simulink model "ServoControlWSpeed_x10"  (R2014a)
settings: Solver=FixedStepDiscrete  StartTime=0.0  StopTime=400000  FixedStep=1  RelTol=1e-3
libraries: hdlsllib x18, simulink x2
settings Model: Creator=schirner  LastModifiedBy=rouan.c
settings DataIOCC: SaveFormat=StructureWithTime
settings OptimizationCC: BlockReduction=off  ConditionallyExecuteInputs=off  InlineParams=on
settings DebuggingCC: AlgebraicLoopMsg=error  MergeDetectMultiDrivingBlocksExec=error
settings HardwareCC: ProdHWDeviceType=ASIC/FPGA->ASIC/FPGA  ProdEqTarget=off

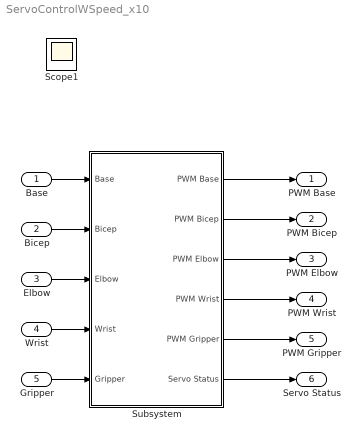
== system ServoControlWSpeed_x10 ==
  Base : Inport  OutDataTypeStr=uint16  SampleTime=1
  Bicep : Inport  Port=2  OutDataTypeStr=uint16  SampleTime=1
  Elbow : Inport  Port=3  OutDataTypeStr=uint16  SampleTime=1
  Wrist : Inport  Port=4  OutDataTypeStr=uint16  SampleTime=1
  Gripper : Inport  Port=5  OutDataTypeStr=uint16  SampleTime=1
  Subsystem : Subsystem  TreatAsAtomicUnit=on  SystemSampleTime=1
  PWM Base : Outport
  PWM Bicep : Outport  Port=2
  PWM Elbow : Outport  Port=3
  PWM Wrist : Outport  Port=4
  PWM Gripper : Outport  Port=5
  Servo Status : Outport  Port=6
  Scope1 : Scope
  wires:
  Subsystem/1(PWM Base) -> PWM Base/1
  Subsystem/2(PWM Bicep) -> PWM Bicep/1
  Subsystem/3(PWM Elbow) -> PWM Elbow/1
  Subsystem/4(PWM Wrist) -> PWM Wrist/1
  Subsystem/5(PWM Gripper) -> PWM Gripper/1
  Subsystem/6("Servo Status ") -> Servo Status/1
  Elbow/1 -> Subsystem/3(Elbow)
  Wrist/1 -> Subsystem/4(Wrist)
  Gripper/1 -> Subsystem/5(Gripper)
  Base/1 -> Subsystem/1(Base)
  Bicep/1 -> Subsystem/2(Bicep)

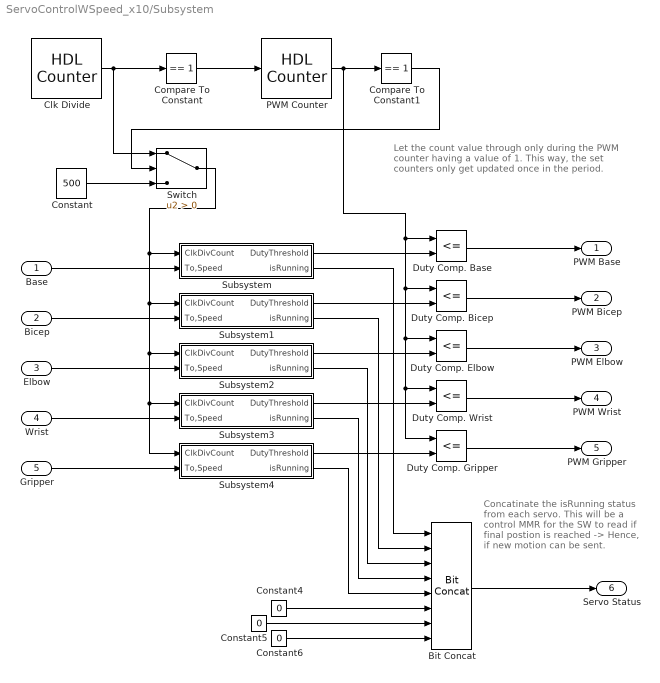
== system ServoControlWSpeed_x10/Subsystem ==
  note: Let the count value through only during
      | the PWM counter having a value of 1.
      | This way, the set counters only get updated
      | once in the period.
  note: Concatinate the isRunning status from each servo. This will be a control MMR for the SW to read if final postion is reached -> Hence, if new motion can be sent.
  Base : Inport  OutDataTypeStr=uint16
  Bicep : Inport  Port=2  OutDataTypeStr=uint16
  Elbow : Inport  Port=3  OutDataTypeStr=uint16
  Wrist : Inport  Port=4  OutDataTypeStr=uint16
  Gripper : Inport  Port=5  OutDataTypeStr=uint16
  Bit Concat : hdlsllib/HDL Operations/Bit Concat  numInputs=8
  Clk Divide : hdlsllib/HDL Operations/HDL Counter  CountType=Count limited  CountInit=1  CountStep=1  CountMax=50  CountFromType=Initial value  CountFrom=1  CountResetPort=off  CountLoadPort=off  CountEnbPort=off  CountDirPort=off  CountDataType=Unsigned  CountWordLen=16  CountFracLen=0  CountSampTime=1
  Compare To Constant : simulink/Logic and Bit Operations/Compare To Constant  relop===  const=1  OutDataTypeStr=boolean
  Compare To Constant1 : simulink/Logic and Bit Operations/Compare To Constant  relop===  const=1  OutDataTypeStr=boolean
  Constant : Constant  Value=500  OutDataTypeStr=int16
  Constant4 : Constant  Value=0  OutDataTypeStr=boolean
  Constant5 : Constant  Value=0  OutDataTypeStr=boolean
  Constant6 : Constant  Value=0  OutDataTypeStr=boolean
  Duty Comp. Base : RelationalOperator  Operator=<=  OutDataTypeStr=boolean
  Duty Comp. Bicep : RelationalOperator  Operator=<=  OutDataTypeStr=boolean
  Duty Comp. Elbow : RelationalOperator  Operator=<=  OutDataTypeStr=boolean
  Duty Comp. Gripper : RelationalOperator  Operator=<=  OutDataTypeStr=boolean
  Duty Comp. Wrist : RelationalOperator  Operator=<=  OutDataTypeStr=boolean
  PWM Counter : hdlsllib/HDL Operations/HDL Counter  CountType=Count limited  CountInit=1  CountStep=1  CountMax=20000  CountFromType=Initial value  CountFrom=1  CountResetPort=off  CountLoadPort=off  CountEnbPort=on  CountDirPort=off  CountDataType=Unsigned  CountWordLen=16  CountFracLen=0  CountSampTime=1
  Subsystem : Subsystem
  Subsystem1 : Subsystem
  Subsystem2 : Subsystem
  Subsystem3 : Subsystem
  Subsystem4 : Subsystem
  Switch : Switch  Criteria=u2 > Threshold
  PWM Base : Outport
  PWM Bicep : Outport  Port=2
  PWM Elbow : Outport  Port=3
  PWM Wrist : Outport  Port=4
  PWM Gripper : Outport  Port=5
  "Servo Status " : Outport  Port=6  OutDataTypeStr=uint8
  wires:
  Duty Comp. Bicep/1 -> PWM Bicep/1
  Compare To Constant/1 -> PWM Counter/1
  Duty Comp. Elbow/1 -> PWM Elbow/1
  Duty Comp. Gripper/1 -> PWM Gripper/1
  Duty Comp. Wrist/1 -> PWM Wrist/1
  PWM Counter/1 -> Duty Comp. Bicep/1, Duty Comp. Gripper/1, Duty Comp. Wrist/1, Duty Comp. Elbow/1, Duty Comp. Base/1, Compare To Constant1/1
  Duty Comp. Base/1 -> PWM Base/1
  Base/1 -> Subsystem/2(To,Speed)
  Subsystem/1(DutyThreshold) -> Duty Comp. Base/2
  Bit Concat/1 -> "Servo Status "/1
  Subsystem/2(isRunning) -> Bit Concat/1
  Constant6/1 -> Bit Concat/8
  Constant5/1 -> Bit Concat/7
  Constant4/1 -> Bit Concat/6
  Bicep/1 -> Subsystem1/2(To,Speed)
  Elbow/1 -> Subsystem2/2(To,Speed)
  Wrist/1 -> Subsystem3/2(To,Speed)
  Gripper/1 -> Subsystem4/2(To,Speed)
  Subsystem1/1(DutyThreshold) -> Duty Comp. Bicep/2
  Subsystem2/1(DutyThreshold) -> Duty Comp. Elbow/2
  Subsystem3/1(DutyThreshold) -> Duty Comp. Wrist/2
  Subsystem4/1(DutyThreshold) -> Duty Comp. Gripper/2
  Subsystem1/2(isRunning) -> Bit Concat/2
  Subsystem2/2(isRunning) -> Bit Concat/3
  Subsystem3/2(isRunning) -> Bit Concat/4
  Subsystem4/2(isRunning) -> Bit Concat/5
  Compare To Constant1/1 -> Switch/2
  Clk Divide/1 -> Switch/1, Compare To Constant/1
  Constant/1 -> Switch/3
  Switch/1 -> Subsystem1/1(ClkDivCount), Subsystem2/1(ClkDivCount), Subsystem4/1(ClkDivCount), Subsystem3/1(ClkDivCount), Subsystem/1(ClkDivCount)

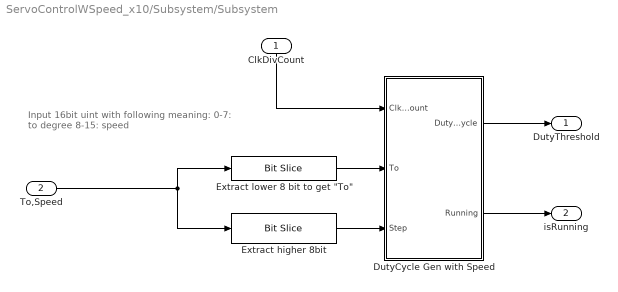
== system ServoControlWSpeed_x10/Subsystem/Subsystem ==
  note: Input 16bit uint with following meaning:
      | 0-7:	to degree
      | 8-15:	speed
  ClkDivCount : Inport
  To,Speed : Inport  Port=2
  DutyCycle Gen with Speed : Subsystem
  Extract higher 8bit : hdlsllib/HDL Operations/Bit Slice  lidx=15  ridx=8
  "Extract lower 8 bit to get \"To\"" : hdlsllib/HDL Operations/Bit Slice  lidx=7  ridx=0
  DutyThreshold : Outport
  isRunning : Outport  Port=2
  wires:
  "Extract lower 8 bit to get \"To\""/1 -> DutyCycle Gen with Speed/2(To)
  ClkDivCount/1 -> DutyCycle Gen with Speed/1(ClkDivCount)
  DutyCycle Gen with Speed/1(Duty Cycle) -> DutyThreshold/1
  To,Speed/1 -> "Extract lower 8 bit to get \"To\""/1, Extract higher 8bit/1
  Extract higher 8bit/1 -> DutyCycle Gen with Speed/3(Step)
  DutyCycle Gen with Speed/2(Running) -> isRunning/1

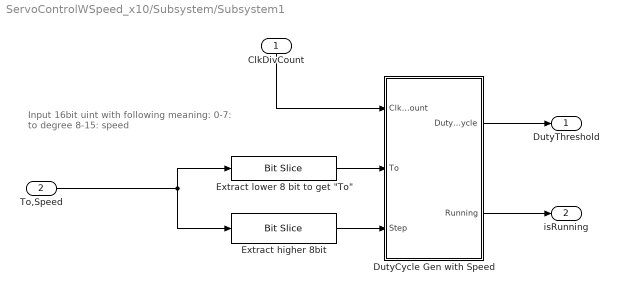
== system ServoControlWSpeed_x10/Subsystem/Subsystem1 ==
  note: Input 16bit uint with following meaning:
      | 0-7:	to degree
      | 8-15:	speed
  ClkDivCount : Inport
  To,Speed : Inport  Port=2
  DutyCycle Gen with Speed : Subsystem
  Extract higher 8bit : hdlsllib/HDL Operations/Bit Slice  lidx=15  ridx=8
  "Extract lower 8 bit to get \"To\"" : hdlsllib/HDL Operations/Bit Slice  lidx=7  ridx=0
  DutyThreshold : Outport
  isRunning : Outport  Port=2
  wires:
  "Extract lower 8 bit to get \"To\""/1 -> DutyCycle Gen with Speed/2(To)
  ClkDivCount/1 -> DutyCycle Gen with Speed/1(ClkDivCount)
  DutyCycle Gen with Speed/1(Duty Cycle) -> DutyThreshold/1
  To,Speed/1 -> "Extract lower 8 bit to get \"To\""/1, Extract higher 8bit/1
  Extract higher 8bit/1 -> DutyCycle Gen with Speed/3(Step)
  DutyCycle Gen with Speed/2(Running) -> isRunning/1

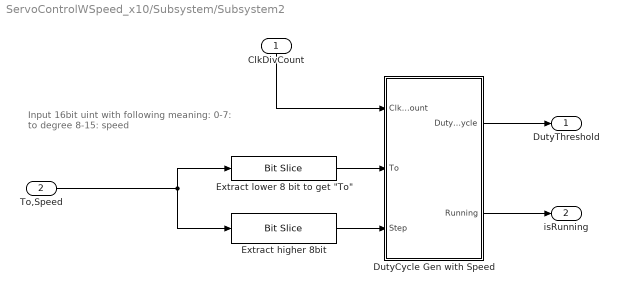
== system ServoControlWSpeed_x10/Subsystem/Subsystem2 ==
  note: Input 16bit uint with following meaning:
      | 0-7:	to degree
      | 8-15:	speed
  ClkDivCount : Inport
  To,Speed : Inport  Port=2
  DutyCycle Gen with Speed : Subsystem
  Extract higher 8bit : hdlsllib/HDL Operations/Bit Slice  lidx=15  ridx=8
  "Extract lower 8 bit to get \"To\"" : hdlsllib/HDL Operations/Bit Slice  lidx=7  ridx=0
  DutyThreshold : Outport
  isRunning : Outport  Port=2
  wires:
  "Extract lower 8 bit to get \"To\""/1 -> DutyCycle Gen with Speed/2(To)
  ClkDivCount/1 -> DutyCycle Gen with Speed/1(ClkDivCount)
  DutyCycle Gen with Speed/1(Duty Cycle) -> DutyThreshold/1
  To,Speed/1 -> "Extract lower 8 bit to get \"To\""/1, Extract higher 8bit/1
  Extract higher 8bit/1 -> DutyCycle Gen with Speed/3(Step)
  DutyCycle Gen with Speed/2(Running) -> isRunning/1

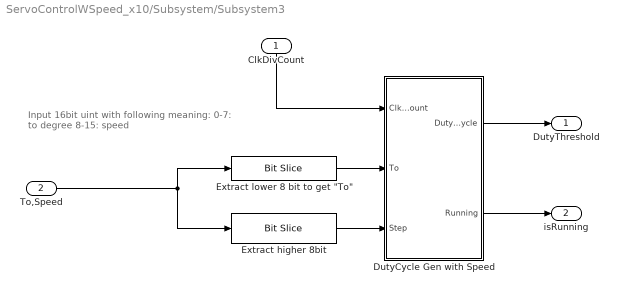
== system ServoControlWSpeed_x10/Subsystem/Subsystem3 ==
  note: Input 16bit uint with following meaning:
      | 0-7:	to degree
      | 8-15:	speed
  ClkDivCount : Inport
  To,Speed : Inport  Port=2
  DutyCycle Gen with Speed : Subsystem
  Extract higher 8bit : hdlsllib/HDL Operations/Bit Slice  lidx=15  ridx=8
  "Extract lower 8 bit to get \"To\"" : hdlsllib/HDL Operations/Bit Slice  lidx=7  ridx=0
  DutyThreshold : Outport
  isRunning : Outport  Port=2
  wires:
  "Extract lower 8 bit to get \"To\""/1 -> DutyCycle Gen with Speed/2(To)
  ClkDivCount/1 -> DutyCycle Gen with Speed/1(ClkDivCount)
  DutyCycle Gen with Speed/1(Duty Cycle) -> DutyThreshold/1
  To,Speed/1 -> "Extract lower 8 bit to get \"To\""/1, Extract higher 8bit/1
  Extract higher 8bit/1 -> DutyCycle Gen with Speed/3(Step)
  DutyCycle Gen with Speed/2(Running) -> isRunning/1

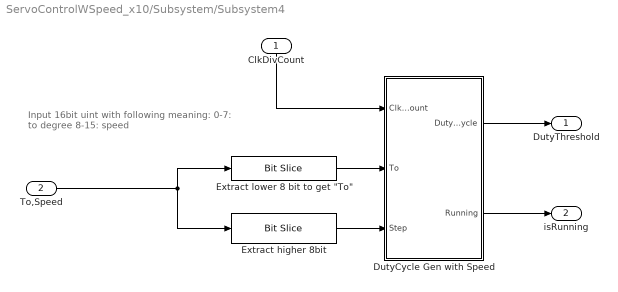
== system ServoControlWSpeed_x10/Subsystem/Subsystem4 ==
  note: Input 16bit uint with following meaning:
      | 0-7:	to degree
      | 8-15:	speed
  ClkDivCount : Inport
  To,Speed : Inport  Port=2
  DutyCycle Gen with Speed : Subsystem
  Extract higher 8bit : hdlsllib/HDL Operations/Bit Slice  lidx=15  ridx=8
  "Extract lower 8 bit to get \"To\"" : hdlsllib/HDL Operations/Bit Slice  lidx=7  ridx=0
  DutyThreshold : Outport
  isRunning : Outport  Port=2
  wires:
  "Extract lower 8 bit to get \"To\""/1 -> DutyCycle Gen with Speed/2(To)
  ClkDivCount/1 -> DutyCycle Gen with Speed/1(ClkDivCount)
  DutyCycle Gen with Speed/1(Duty Cycle) -> DutyThreshold/1
  To,Speed/1 -> "Extract lower 8 bit to get \"To\""/1, Extract higher 8bit/1
  Extract higher 8bit/1 -> DutyCycle Gen with Speed/3(Step)
  DutyCycle Gen with Speed/2(Running) -> isRunning/1

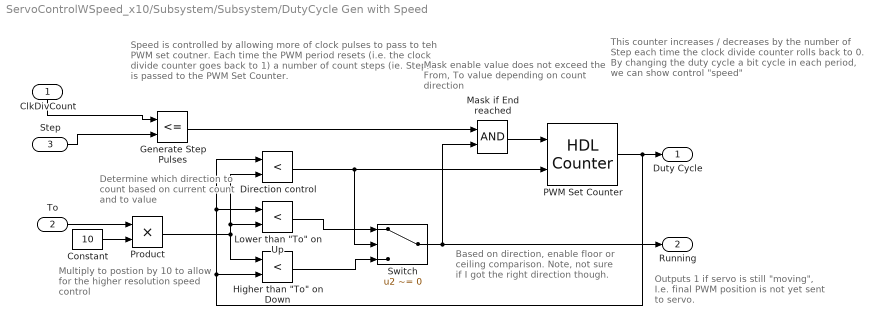
== system ServoControlWSpeed_x10/Subsystem/Subsystem/DutyCycle Gen with Speed ==
  note: Multiply to postion by 10 to
      | allow for the higher resolution
      | speed control
  note: Outputs 1 if servo is still "moving", I.e. final PWM position is not yet sent to servo.
  note: Based on direction, enable floor or ceiling comparison.
      | Note, not sure if I got the right direction though.
  note: This counter increases / decreases by the number of Step each time the clock divide counter rolls back to 0. By changing the duty cycle a bit cycle in each period, we can show control "speed"
  note: Speed is controlled by allowing more
      | of clock pulses to pass to teh PWM set coutner.
      | Each time the PWM period resets (i.e. the clock divide
      | counter goes back to 1) a number of count steps (ie. Steps)
      | is passed to the PWM Set Counter.
  note: Determine which
      | direction to count
      | based on current count and to value
  note: Mask  enable value does
      | not exceed the From, To value
      | depending on count direction
  ClkDivCount : Inport
  To : Inport  Port=2  OutDataTypeStr=uint8
  Step : Inport  Port=3  OutDataTypeStr=uint8
  Constant : Constant  Value=10  OutDataTypeStr=uint8  SampleTime=Inf
  Direction control : RelationalOperator  Operator=<  OutDataTypeStr=boolean
  Generate Step Pulses : RelationalOperator  Operator=<=  OutDataTypeStr=boolean
  "Higher than \"To\" on Down" : RelationalOperator  Operator=<  OutDataTypeStr=boolean
  "Lower than \"To\" on Up" : RelationalOperator  Operator=<  OutDataTypeStr=boolean
  Mask if End reached : Logic  AllPortsSameDT=off  OutDataTypeStr=boolean
  PWM Set Counter : hdlsllib/HDL Operations/HDL Counter  CountType=Free running  CountInit=1500  CountStep=1  CountMax=256  CountFromType=Initial value  CountFrom=1500  CountResetPort=off  CountLoadPort=off  CountEnbPort=on  CountDirPort=on  CountDataType=Unsigned  CountWordLen=16  CountFracLen=0  CountSampTime=1
  Product : Product  OutDataTypeStr=uint16
  Switch : Switch  Criteria=u2 ~= 0
  Duty Cycle : Outport
  Running : Outport  Port=2
  wires:
  Generate Step Pulses/1 -> Mask if End reached/1
  PWM Set Counter/1 -> Duty Cycle/1, Direction control/1, "Lower than \"To\" on Up"/1, "Higher than \"To\" on Down"/2
  ClkDivCount/1 -> Generate Step Pulses/1
  Step/1 -> Generate Step Pulses/2
  Product/1 -> Direction control/2, "Lower than \"To\" on Up"/2, "Higher than \"To\" on Down"/1
  Mask if End reached/1 -> PWM Set Counter/1
  Switch/1 -> Running/1, Mask if End reached/2
  Direction control/1 -> Switch/2, PWM Set Counter/2
  "Higher than \"To\" on Down"/1 -> Switch/3
  "Lower than \"To\" on Up"/1 -> Switch/1
  Constant/1 -> Product/2
  To/1 -> Product/1

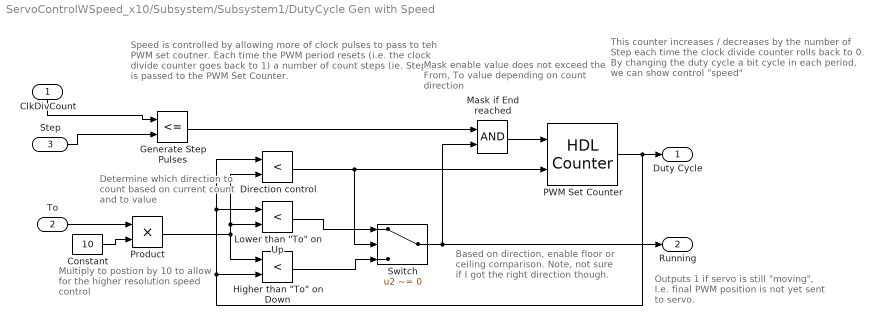
== system ServoControlWSpeed_x10/Subsystem/Subsystem1/DutyCycle Gen with Speed ==
  note: Multiply to postion by 10 to
      | allow for the higher resolution
      | speed control
  note: Outputs 1 if servo is still "moving", I.e. final PWM position is not yet sent to servo.
  note: Based on direction, enable floor or ceiling comparison.
      | Note, not sure if I got the right direction though.
  note: This counter increases / decreases by the number of Step each time the clock divide counter rolls back to 0. By changing the duty cycle a bit cycle in each period, we can show control "speed"
  note: Speed is controlled by allowing more
      | of clock pulses to pass to teh PWM set coutner.
      | Each time the PWM period resets (i.e. the clock divide
      | counter goes back to 1) a number of count steps (ie. Steps)
      | is passed to the PWM Set Counter.
  note: Determine which
      | direction to count
      | based on current count and to value
  note: Mask  enable value does
      | not exceed the From, To value
      | depending on count direction
  ClkDivCount : Inport
  To : Inport  Port=2  OutDataTypeStr=uint8
  Step : Inport  Port=3  OutDataTypeStr=uint8
  Constant : Constant  Value=10  OutDataTypeStr=uint8  SampleTime=Inf
  Direction control : RelationalOperator  Operator=<  OutDataTypeStr=boolean
  Generate Step Pulses : RelationalOperator  Operator=<=  OutDataTypeStr=boolean
  "Higher than \"To\" on Down" : RelationalOperator  Operator=<  OutDataTypeStr=boolean
  "Lower than \"To\" on Up" : RelationalOperator  Operator=<  OutDataTypeStr=boolean
  Mask if End reached : Logic  AllPortsSameDT=off  OutDataTypeStr=boolean
  PWM Set Counter : hdlsllib/HDL Operations/HDL Counter  CountType=Free running  CountInit=1500  CountStep=1  CountMax=256  CountFromType=Initial value  CountFrom=1500  CountResetPort=off  CountLoadPort=off  CountEnbPort=on  CountDirPort=on  CountDataType=Unsigned  CountWordLen=16  CountFracLen=0  CountSampTime=1
  Product : Product  OutDataTypeStr=uint16
  Switch : Switch  Criteria=u2 ~= 0
  Duty Cycle : Outport
  Running : Outport  Port=2
  wires:
  Generate Step Pulses/1 -> Mask if End reached/1
  PWM Set Counter/1 -> Duty Cycle/1, Direction control/1, "Lower than \"To\" on Up"/1, "Higher than \"To\" on Down"/2
  ClkDivCount/1 -> Generate Step Pulses/1
  Step/1 -> Generate Step Pulses/2
  Product/1 -> Direction control/2, "Lower than \"To\" on Up"/2, "Higher than \"To\" on Down"/1
  Mask if End reached/1 -> PWM Set Counter/1
  Switch/1 -> Running/1, Mask if End reached/2
  Direction control/1 -> Switch/2, PWM Set Counter/2
  "Higher than \"To\" on Down"/1 -> Switch/3
  "Lower than \"To\" on Up"/1 -> Switch/1
  Constant/1 -> Product/2
  To/1 -> Product/1

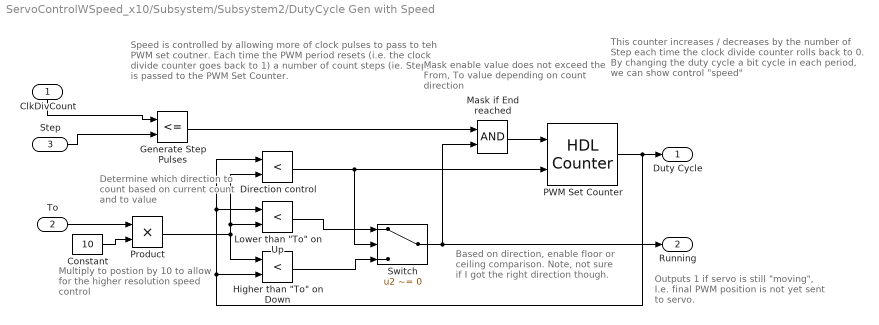
== system ServoControlWSpeed_x10/Subsystem/Subsystem2/DutyCycle Gen with Speed ==
  note: Multiply to postion by 10 to
      | allow for the higher resolution
      | speed control
  note: Outputs 1 if servo is still "moving", I.e. final PWM position is not yet sent to servo.
  note: Based on direction, enable floor or ceiling comparison.
      | Note, not sure if I got the right direction though.
  note: This counter increases / decreases by the number of Step each time the clock divide counter rolls back to 0. By changing the duty cycle a bit cycle in each period, we can show control "speed"
  note: Speed is controlled by allowing more
      | of clock pulses to pass to teh PWM set coutner.
      | Each time the PWM period resets (i.e. the clock divide
      | counter goes back to 1) a number of count steps (ie. Steps)
      | is passed to the PWM Set Counter.
  note: Determine which
      | direction to count
      | based on current count and to value
  note: Mask  enable value does
      | not exceed the From, To value
      | depending on count direction
  ClkDivCount : Inport
  To : Inport  Port=2  OutDataTypeStr=uint8
  Step : Inport  Port=3  OutDataTypeStr=uint8
  Constant : Constant  Value=10  OutDataTypeStr=uint8  SampleTime=Inf
  Direction control : RelationalOperator  Operator=<  OutDataTypeStr=boolean
  Generate Step Pulses : RelationalOperator  Operator=<=  OutDataTypeStr=boolean
  "Higher than \"To\" on Down" : RelationalOperator  Operator=<  OutDataTypeStr=boolean
  "Lower than \"To\" on Up" : RelationalOperator  Operator=<  OutDataTypeStr=boolean
  Mask if End reached : Logic  AllPortsSameDT=off  OutDataTypeStr=boolean
  PWM Set Counter : hdlsllib/HDL Operations/HDL Counter  CountType=Free running  CountInit=1500  CountStep=1  CountMax=256  CountFromType=Initial value  CountFrom=1500  CountResetPort=off  CountLoadPort=off  CountEnbPort=on  CountDirPort=on  CountDataType=Unsigned  CountWordLen=16  CountFracLen=0  CountSampTime=1
  Product : Product  OutDataTypeStr=uint16
  Switch : Switch  Criteria=u2 ~= 0
  Duty Cycle : Outport
  Running : Outport  Port=2
  wires:
  Generate Step Pulses/1 -> Mask if End reached/1
  PWM Set Counter/1 -> Duty Cycle/1, Direction control/1, "Lower than \"To\" on Up"/1, "Higher than \"To\" on Down"/2
  ClkDivCount/1 -> Generate Step Pulses/1
  Step/1 -> Generate Step Pulses/2
  Product/1 -> Direction control/2, "Lower than \"To\" on Up"/2, "Higher than \"To\" on Down"/1
  Mask if End reached/1 -> PWM Set Counter/1
  Switch/1 -> Running/1, Mask if End reached/2
  Direction control/1 -> Switch/2, PWM Set Counter/2
  "Higher than \"To\" on Down"/1 -> Switch/3
  "Lower than \"To\" on Up"/1 -> Switch/1
  Constant/1 -> Product/2
  To/1 -> Product/1

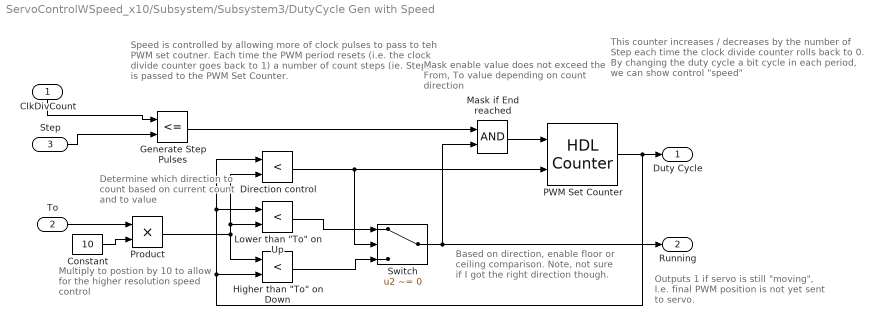
== system ServoControlWSpeed_x10/Subsystem/Subsystem3/DutyCycle Gen with Speed ==
  note: Multiply to postion by 10 to
      | allow for the higher resolution
      | speed control
  note: Outputs 1 if servo is still "moving", I.e. final PWM position is not yet sent to servo.
  note: Based on direction, enable floor or ceiling comparison.
      | Note, not sure if I got the right direction though.
  note: This counter increases / decreases by the number of Step each time the clock divide counter rolls back to 0. By changing the duty cycle a bit cycle in each period, we can show control "speed"
  note: Speed is controlled by allowing more
      | of clock pulses to pass to teh PWM set coutner.
      | Each time the PWM period resets (i.e. the clock divide
      | counter goes back to 1) a number of count steps (ie. Steps)
      | is passed to the PWM Set Counter.
  note: Determine which
      | direction to count
      | based on current count and to value
  note: Mask  enable value does
      | not exceed the From, To value
      | depending on count direction
  ClkDivCount : Inport
  To : Inport  Port=2  OutDataTypeStr=uint8
  Step : Inport  Port=3  OutDataTypeStr=uint8
  Constant : Constant  Value=10  OutDataTypeStr=uint8  SampleTime=Inf
  Direction control : RelationalOperator  Operator=<  OutDataTypeStr=boolean
  Generate Step Pulses : RelationalOperator  Operator=<=  OutDataTypeStr=boolean
  "Higher than \"To\" on Down" : RelationalOperator  Operator=<  OutDataTypeStr=boolean
  "Lower than \"To\" on Up" : RelationalOperator  Operator=<  OutDataTypeStr=boolean
  Mask if End reached : Logic  AllPortsSameDT=off  OutDataTypeStr=boolean
  PWM Set Counter : hdlsllib/HDL Operations/HDL Counter  CountType=Free running  CountInit=1500  CountStep=1  CountMax=256  CountFromType=Initial value  CountFrom=1500  CountResetPort=off  CountLoadPort=off  CountEnbPort=on  CountDirPort=on  CountDataType=Unsigned  CountWordLen=16  CountFracLen=0  CountSampTime=1
  Product : Product  OutDataTypeStr=uint16
  Switch : Switch  Criteria=u2 ~= 0
  Duty Cycle : Outport
  Running : Outport  Port=2
  wires:
  Generate Step Pulses/1 -> Mask if End reached/1
  PWM Set Counter/1 -> Duty Cycle/1, Direction control/1, "Lower than \"To\" on Up"/1, "Higher than \"To\" on Down"/2
  ClkDivCount/1 -> Generate Step Pulses/1
  Step/1 -> Generate Step Pulses/2
  Product/1 -> Direction control/2, "Lower than \"To\" on Up"/2, "Higher than \"To\" on Down"/1
  Mask if End reached/1 -> PWM Set Counter/1
  Switch/1 -> Running/1, Mask if End reached/2
  Direction control/1 -> Switch/2, PWM Set Counter/2
  "Higher than \"To\" on Down"/1 -> Switch/3
  "Lower than \"To\" on Up"/1 -> Switch/1
  Constant/1 -> Product/2
  To/1 -> Product/1

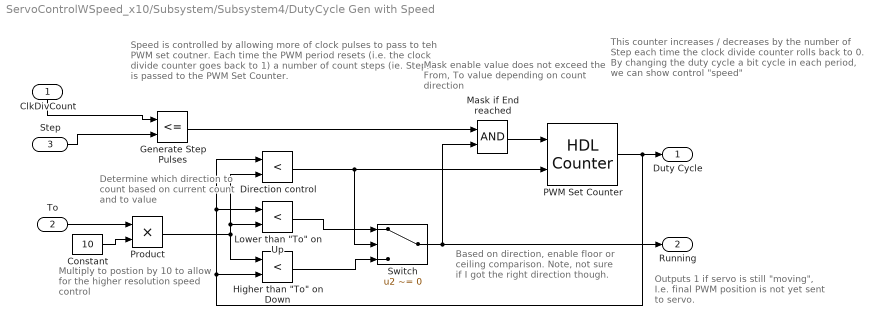
== system ServoControlWSpeed_x10/Subsystem/Subsystem4/DutyCycle Gen with Speed ==
  note: Multiply to postion by 10 to
      | allow for the higher resolution
      | speed control
  note: Outputs 1 if servo is still "moving", I.e. final PWM position is not yet sent to servo.
  note: Based on direction, enable floor or ceiling comparison.
      | Note, not sure if I got the right direction though.
  note: This counter increases / decreases by the number of Step each time the clock divide counter rolls back to 0. By changing the duty cycle a bit cycle in each period, we can show control "speed"
  note: Speed is controlled by allowing more
      | of clock pulses to pass to teh PWM set coutner.
      | Each time the PWM period resets (i.e. the clock divide
      | counter goes back to 1) a number of count steps (ie. Steps)
      | is passed to the PWM Set Counter.
  note: Determine which
      | direction to count
      | based on current count and to value
  note: Mask  enable value does
      | not exceed the From, To value
      | depending on count direction
  ClkDivCount : Inport
  To : Inport  Port=2  OutDataTypeStr=uint8
  Step : Inport  Port=3  OutDataTypeStr=uint8
  Constant : Constant  Value=10  OutDataTypeStr=uint8  SampleTime=Inf
  Direction control : RelationalOperator  Operator=<  OutDataTypeStr=boolean
  Generate Step Pulses : RelationalOperator  Operator=<=  OutDataTypeStr=boolean
  "Higher than \"To\" on Down" : RelationalOperator  Operator=<  OutDataTypeStr=boolean
  "Lower than \"To\" on Up" : RelationalOperator  Operator=<  OutDataTypeStr=boolean
  Mask if End reached : Logic  AllPortsSameDT=off  OutDataTypeStr=boolean
  PWM Set Counter : hdlsllib/HDL Operations/HDL Counter  CountType=Free running  CountInit=1500  CountStep=1  CountMax=256  CountFromType=Initial value  CountFrom=1500  CountResetPort=off  CountLoadPort=off  CountEnbPort=on  CountDirPort=on  CountDataType=Unsigned  CountWordLen=16  CountFracLen=0  CountSampTime=1
  Product : Product  OutDataTypeStr=uint16
  Switch : Switch  Criteria=u2 ~= 0
  Duty Cycle : Outport
  Running : Outport  Port=2
  wires:
  Generate Step Pulses/1 -> Mask if End reached/1
  PWM Set Counter/1 -> Duty Cycle/1, Direction control/1, "Lower than \"To\" on Up"/1, "Higher than \"To\" on Down"/2
  ClkDivCount/1 -> Generate Step Pulses/1
  Step/1 -> Generate Step Pulses/2
  Product/1 -> Direction control/2, "Lower than \"To\" on Up"/2, "Higher than \"To\" on Down"/1
  Mask if End reached/1 -> PWM Set Counter/1
  Switch/1 -> Running/1, Mask if End reached/2
  Direction control/1 -> Switch/2, PWM Set Counter/2
  "Higher than \"To\" on Down"/1 -> Switch/3
  "Lower than \"To\" on Up"/1 -> Switch/1
  Constant/1 -> Product/2
  To/1 -> Product/1
